simulink model "explore"  (Simulink 8.3)
settings: Solver=ode4  StartTime=0.0  StopTime=600  FixedStep=0.001  RelTol=1e-3
PostLoadFcn:
  | , if any(exist('dsrtsu_mdlpostloadfcn', 'file') == [2, 3, 6]), try dsrtsu_mdlpostloadfcn('Execute', bdroot); catch fprintf('Error in PostLoadFcn (dsrtsu_mdlpostloadfcn) for model "%s":\n %s\n', bdroot, lasterr); end, end,
values from neighbouring files (symbols this model uses):
  A = kron(eye(2),A)    [explore_setup.m]
  Ae = Ah    [explore_setup.m]
  Av = [0 1 0; zeros(2,1) Av]    [explore_setup.m]
  Aw = [0 1; 0 Aw]    [explore_setup.m]
  B = kron(eye(2),B)    [explore_setup.m]
  Be = Bh    [explore_setup.m]
  Bv = [0; Bv]    [explore_setup.m]
  Bw = [0; Bw*Cw]    [explore_setup.m]
  Ce = Ch    [explore_setup.m]
  Cv = [1 0 0]    [explore_setup.m]
  Cw = [1 0]    [explore_setup.m]
  dt = 0.15    [explore_setup.m]
  Fu = kron(eye(2), Fu)    [explore_setup.m]
  Fus = kron(eye(2), Fus)    [explore_setup.m]
  Fx = kron(eye(2),Fx)    [explore_setup.m]
  Fxf = 1e-6*eye(8)    [explore_setup.m]
  Fxs = kron(eye(2),Fxs)    [explore_setup.m]
  goal = [1.8750    1.5000]    [explore_setup.m]    (also in visualizeSim.m = u(169:170))
  homePos = [-2.5 -1]    [explore_setup.m]
  Le = place(Ae', Ce', -[3.1 3.0 3.2])'    [explore_setup.m]
  Lv = place(Av', Cv', -[3.1 3.0 3.2])'    [explore_setup.m]
  Lw = place(Aw', Cw', -[3.1 3.0])'    [explore_setup.m]
  nodeV0 = (1/.4)*sqrt((nodeX-goal(1)).*(nodeX-goal(1))+(nodeY-goal(2)).*(nodeY-goal(2)))    [explore_setup.m]
  nodeX = [goal(1); nodeX]    [explore_setup.m]
  nodeY = [goal(2); nodeY]    [explore_setup.m]
  obst = [-2.4950    1.5000    1.3750    2.0000 ... (first row only)    [explore_setup.m]    (also in visualizeSim.m = reshape(obstIn,4,nObst)')
  Q = diag([5 5 5 2 5 5 5 2])    [explore_setup.m]
  Qf = diag([5 5 5 2 5 5 5 2])    [explore_setup.m]
  R = diag([10 10])    [explore_setup.m]
  T = 16    [explore_setup.m]
undefined symbols (not defined in the file or in its folder): bd, bx, C, Ef_block, g, gt, H, hc, hcs, hp, hps, hx, hxs, P, Ps
undefined symbols (not defined in the file): Ed, ef, Exf, f, ff, Fp, Fpf, Fps, fs, q, qf, r
libraries: simulink x1
settings Model: DSRTSU_INTERNAL_RTI_VER=400  DSRTSU_INTERNAL_RTI_TYPE=rti1401  Creator=aeagr  LastModifiedBy=aeagr  BufferReuse=off
settings OptimizationCC: BlockReduction=off  OptimizeBlockIOStorage=off  BufferReuse=off  GlobalBufferReuse=off  ExpressionFolding=off  ExpressionDepthLimit=2147483647  LocalBlockOutputs=off  SimCompilerOptimization=On
settings DebuggingCC: FcnCallInpInsideContextMsg=UseLocalSettings
settings HardwareCC: ProdIntDivRoundTo=Zero  ProdEndianess=BigEndian  ProdHWDeviceType=Generic->Custom  TargetIntDivRoundTo=Zero  TargetEndianess=BigEndian  TargetHWDeviceType=Generic->Custom
settings RTWCC: ProcessScript=grt_make_rtw_hook
settings GRTTargetCC: CombineOutputUpdateFcns=on  GRTInterface=off

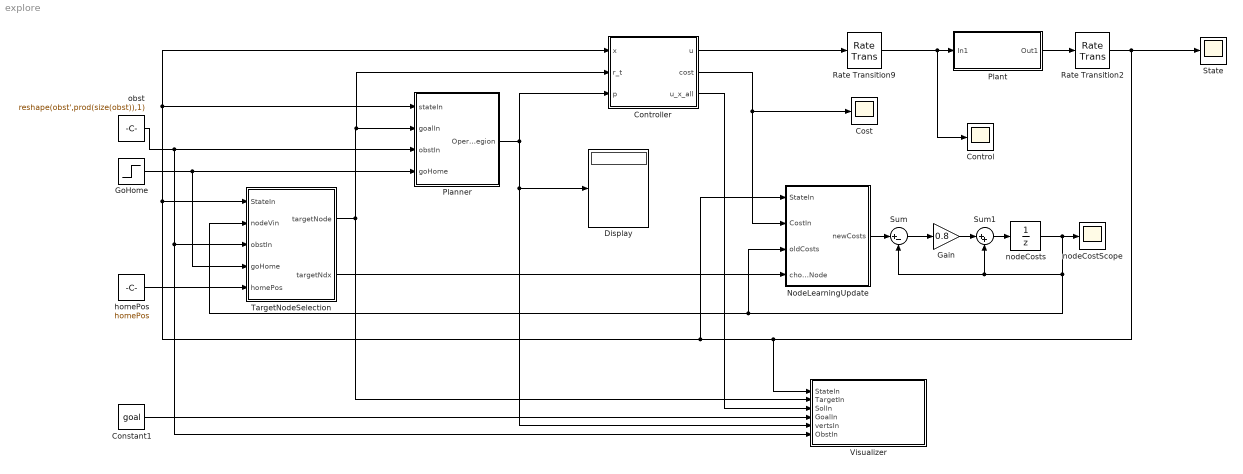
== system explore ==
  Constant1 : Constant  Value=goal
  Control : Scope
      settings: TimeRange=120  YMin=-0.05  YMax=0.12
  Controller : Subsystem  TreatAsAtomicUnit=on  SystemSampleTime=dt
  Cost : Scope
      settings: TimeRange=120  YMin=0  YMax=350  SaveName=ScopeData8
  Display : Display
  Gain : Gain  Gain=0.8
  GoHome : Step  Time=10  Before=1  After=0  SampleTime=dt
  NodeLearningUpdate : Subsystem  TreatAsAtomicUnit=on  SystemSampleTime=dt
  Planner : Subsystem  TreatAsAtomicUnit=on  SystemSampleTime=dt
  Plant : Subsystem
  Rate Transition2 : RateTransition  Integrity=off  OutPortSampleTimeOpt=Inherit  OutPortSampleTime=dt
  Rate Transition9 : RateTransition  Integrity=off  OutPortSampleTimeOpt=Inherit  OutPortSampleTime=dt
  State : Scope
      settings: TimeRange=60  YMin=-200  YMax=225
  Sum : Sum  Inputs=|+-
  Sum1 : Sum  Inputs=|++
  TargetNodeSelection : Subsystem  TreatAsAtomicUnit=on  SystemSampleTime=dt
  Visualizer : Subsystem
  homePos : Constant  Value=homePos
  nodeCostScope : Scope
      settings: TimeRange=120  YMin=0  YMax=19  SaveName=ScopeData2
  nodeCosts : UnitDelay  InitialCondition=nodeV0  SampleTime=dt
  obst : Constant  Value=reshape(obst',prod(size(obst)),1)
  wires:
  Plant/1(Out1) -> Rate Transition2/1
  Planner/1(Operating Region) -> Controller/3(p), Display/1, Visualizer/5(vertsIn)
  Controller/1(u) -> Rate Transition9/1
  Controller/3(u_x_all) -> Visualizer/3(SolIn)
  Constant1/1 -> Visualizer/4(GoalIn)
  obst/1 -> Planner/3(obstIn), Visualizer/6(ObstIn), TargetNodeSelection/3(obstIn)
  TargetNodeSelection/1(targetNode) -> Visualizer/2(TargetIn), Controller/2(r_t), Planner/2(goalIn)
  GoHome/1 -> TargetNodeSelection/4(goHome), Planner/4(goHome)
  Rate Transition9/1 -> Plant/1(In1), Control/1
  Controller/2(cost) -> NodeLearningUpdate/2(CostIn), Cost/1
  Rate Transition2/1 -> State/1, Visualizer/1(StateIn), NodeLearningUpdate/1(StateIn), TargetNodeSelection/1(StateIn), Controller/1(x), Planner/1(stateIn)
  TargetNodeSelection/2(targetNdx) -> NodeLearningUpdate/4(chosenNode)
  nodeCosts/1 -> nodeCostScope/1, TargetNodeSelection/2(nodeVin), NodeLearningUpdate/3(oldCosts), Sum1/2, Sum/2
  homePos/1 -> TargetNodeSelection/5(homePos)
  NodeLearningUpdate/1(newCosts) -> Sum/1
  Sum1/1 -> nodeCosts/1
  Sum/1 -> Gain/1
  Gain/1 -> Sum1/1

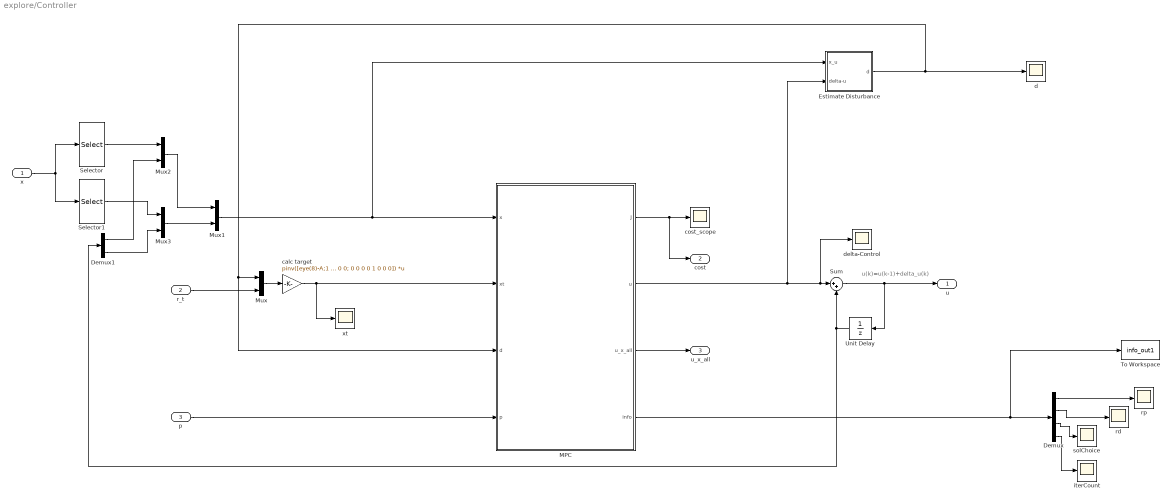
== system explore/Controller ==
  note: u(k)=u(k-1)+delta_u(k)
  x : Inport
  r_t : Inport  Port=2
  p : Inport  Port=3
  Demux : Demux
  Demux1 : Demux  Outputs=2
  Estimate Disturbance : Subsystem
  MPC : Subsystem  TreatAsAtomicUnit=on  mask{A=A, B=B, T=T, dt=-1, Q=Q, R=R, Qf=Qf, qv=q, rv=r, qfv=qf, Fx=Fx, Fu=Fu, Fp=Fp, f=f, Fxs=Fxs, Fus=Fus, Fps=Fps, fs=fs, Fxf=Fxf, Fpf=Fpf, ff=ff, Ef=Exf, Ed=Ed, e=ef, consAllBox=on, numNewton=4, kappa=0.005}
      mask prompts: T "Horizon length T"; dt "Time step"; qv "q"; rv "r"; qfv "qf"; e "ef"; consAllBox "Box constraints"; numNewton "Number of Newton Iterations"; kappa "Barrier weight kappa"
      mask init:
      | % build the big matrices
      | [H,g,gt,P,hx,hc,C,bx,bd,Ps,hxs,hcs,Ef_block,Ed_block,ef_block,hp,hps] = buildmatrices(A,B,Q,R,qv,rv,Qf,qfv,T,Fx,Fu,f,Fxs,Fus,fs,Fxf,ff,Ef,e,Ed,Fp,Fps,Fpf);
      | 
      | % options
      | opts=[];
      | disp(consAllBox)
      | if consAllBox,
      |     opts(1)=1; % 1 = assume diagonal Phi when solving
      | else
      |     opts(1)=0;
      | end
      | opts(2)=numNewton; % Newton iterations
      | opts(3)=1; % 1 = use soft constraints
      | opts(4)=0; % 1 = checking on
      | opts(7)=kappa; % tuning of barrier weight kappa
  Mux{,1..3} (4 alike) : Mux  Inputs=2
  Selector : Selector  InputPortWidth=6  Indices=[1 2 3]
  Selector1 : Selector  InputPortWidth=6  Indices=[1 2 3]+3
  Sum : Sum  Inputs=|++
  To Workspace : ToWorkspace  VariableName=info_out1  SampleTime=-1
  Unit Delay : UnitDelay  SampleTime=-1
  calc target : Gain  Gain=pinv([eye(8)-A;1 0 0 0 0 0 0 0; 0 0 0 0 1 0 0 0])  Multiplication=Matrix(K*u)
  cost_scope : Scope
      settings: YMin=-0.25  YMax=2.5  SaveName=ScopeData10
  d : Scope
      settings: YMin=-0.00025  YMax=0.002  SaveName=ScopeData11
  delta-Control : Scope
      settings: TimeRange=240  YMin=-0.4  YMax=0.35  SaveName=ScopeData2
  iterCount : Scope
      settings: TimeRange=200  YMin=0  YMax=25  SaveName=ScopeData12
  rd : Scope
      settings: YMin=0  YMax=13  SaveName=ScopeData13
  rp : Scope
      settings: YMin=1.65436e-24  YMax=2.75e-08  SaveName=ScopeData14
  solChoice : Scope
      settings: YMin=0.95  YMax=1.05  SaveName=ScopeData15
  xt : Scope
      settings: YMin=-0.25  YMax=2.5  SaveName=ScopeData16
  u : Outport
  cost : Outport  Port=2
  u_x_all : Outport  Port=3
  wires:
  Sum/1 -> u/1, Unit Delay/1
  MPC/2(u) -> Sum/1, delta-Control/1, Estimate Disturbance/2(delta-u)
  Unit Delay/1 -> Demux1/1, Sum/2
  Mux1/1 -> MPC/1(x), Estimate Disturbance/1(x_u)
  Demux/1 -> rp/1
  Demux/2 -> rd/1
  Demux/3 -> solChoice/1
  Estimate Disturbance/1(d) -> MPC/3(d), Mux/1, d/1
  Mux/1 -> calc target/1
  r_t/1 -> Mux/2
  calc target/1 -> MPC/2(xt), xt/1
  Demux/4 -> iterCount/1
  MPC/4(info) -> To Workspace/1, Demux/1
  p/1 -> MPC/4(p)
  MPC/1(J) -> cost/1, cost_scope/1
  MPC/3(u_x_all) -> u_x_all/1
  x/1 -> Selector1/1, Selector/1
  Selector/1 -> Mux2/1
  Selector1/1 -> Mux3/1
  Demux1/1 -> Mux2/2
  Demux1/2 -> Mux3/2
  Mux3/1 -> Mux1/2
  Mux2/1 -> Mux1/1

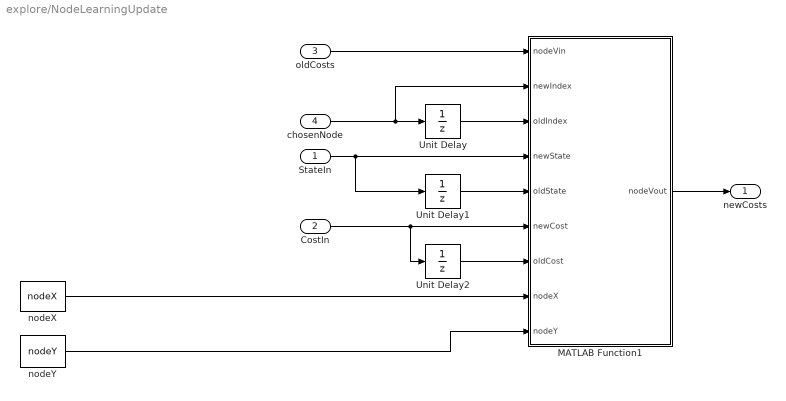
== system explore/NodeLearningUpdate ==
  StateIn : Inport
  CostIn : Inport  Port=2
  oldCosts : Inport  Port=3
  chosenNode : Inport  Port=4
  MATLAB Function1 : MATLAB Function  TreatAsAtomicUnit=on
  Unit Delay : UnitDelay  SampleTime=-1
  Unit Delay1 : UnitDelay  SampleTime=-1
  Unit Delay2 : UnitDelay  SampleTime=-1
  nodeX : Constant  Value=nodeX
  nodeY : Constant  Value=nodeY
  newCosts : Outport
  wires:
  CostIn/1 -> Unit Delay2/1, MATLAB Function1/6(newCost)
  StateIn/1 -> MATLAB Function1/4(newState), Unit Delay1/1
  nodeY/1 -> MATLAB Function1/9(nodeY)
  nodeX/1 -> MATLAB Function1/8(nodeX)
  Unit Delay2/1 -> MATLAB Function1/7(oldCost)
  Unit Delay1/1 -> MATLAB Function1/5(oldState)
  chosenNode/1 -> MATLAB Function1/2(newIndex), Unit Delay/1
  Unit Delay/1 -> MATLAB Function1/3(oldIndex)
  MATLAB Function1/1(nodeVout) -> newCosts/1
  oldCosts/1 -> MATLAB Function1/1(nodeVin)

== system explore/Planner ==
  stateIn : Inport
  goalIn : Inport  Port=2
  obstIn : Inport  Port=3
  goHome : Inport  Port=4
  MATLAB Function : MATLAB Function  TreatAsAtomicUnit=on
  Operating Region : Outport
  wires:
  stateIn/1 -> MATLAB Function/1(state)
  goHome/1 -> MATLAB Function/2(goHome)
  MATLAB Function/1(verts) -> Operating Region/1
  goalIn/1 -> MATLAB Function/4(goal)
  obstIn/1 -> MATLAB Function/3(obst)

== system explore/Plant ==
  In1 : Inport
  AR.Drone : Subsystem
  Demux1 : Demux  Outputs=2
  Fixed point hold : Subsystem
  Mux : Mux  Inputs=3
  Other inputs : Selector  InputPortWidth=4  Indices=[3 4]
  "Position, Velocity" : Selector  InputPortWidth=11  Indices=[1 4 7 10 2 5 8 11]
  Select Gxy : Selector  InputPortWidth=11  Indices=[1 2 3 4 5 6]
  Out1 : Outport
  wires:
  Other inputs/1 -> Demux1/1
  Mux/1 -> AR.Drone/1(U Global)
  Fixed point hold/1(U Global) -> Other inputs/1
  "Position, Velocity"/1 -> Fixed point hold/1(X Global)
  AR.Drone/1(X Global) -> "Position, Velocity"/1, Select Gxy/1
  Select Gxy/1 -> Out1/1
  In1/1 -> Mux/1
  Demux1/1 -> Mux/2
  Demux1/2 -> Mux/3

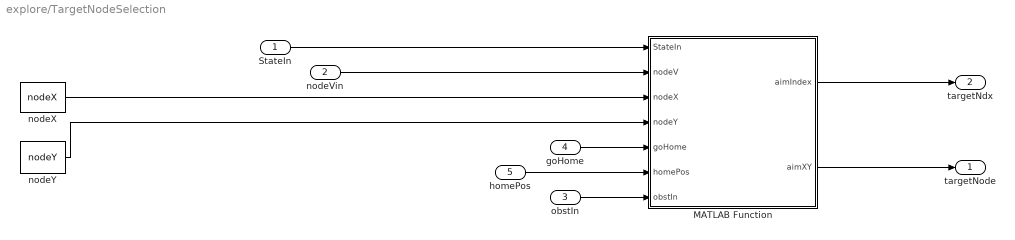
== system explore/TargetNodeSelection ==
  StateIn : Inport
  nodeVin : Inport  Port=2
  obstIn : Inport  Port=3
  goHome : Inport  Port=4
  homePos : Inport  Port=5
  MATLAB Function : MATLAB Function  TreatAsAtomicUnit=on  SystemSampleTime=dt
  nodeX : Constant  Value=nodeX
  nodeY : Constant  Value=nodeY
  targetNode : Outport
  targetNdx : Outport  Port=2
  wires:
  nodeX/1 -> MATLAB Function/3(nodeX)
  nodeY/1 -> MATLAB Function/4(nodeY)
  StateIn/1 -> MATLAB Function/1(StateIn)
  MATLAB Function/2(aimXY) -> targetNode/1
  goHome/1 -> MATLAB Function/5(goHome)
  obstIn/1 -> MATLAB Function/7(obstIn)
  MATLAB Function/1(aimIndex) -> targetNdx/1
  nodeVin/1 -> MATLAB Function/2(nodeV)
  homePos/1 -> MATLAB Function/6(homePos)

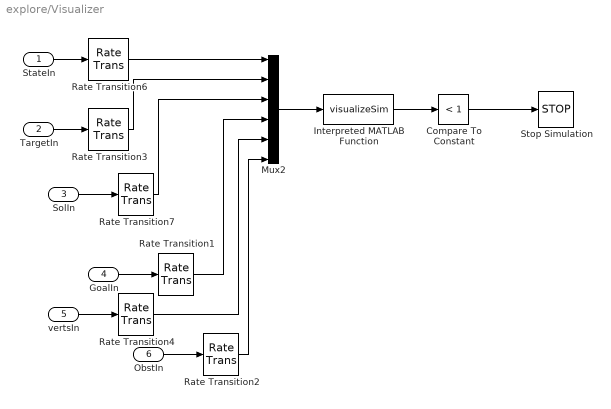
== system explore/Visualizer ==
  StateIn : Inport
  TargetIn : Inport  Port=2
  SolIn : Inport  Port=3
  GoalIn : Inport  Port=4
  vertsIn : Inport  Port=5
  ObstIn : Inport  Port=6
  Compare To Constant : simulink/Logic and Bit Operations/Compare To Constant  relop=<  const=1  OutDataTypeStr=boolean
  Interpreted MATLAB Function : MATLABFcn  MATLABFcn=visualizeSim
  Mux2 : Mux  Inputs=6
  Rate Transition{1..4,6..7} (6 alike) : RateTransition  Integrity=off  OutPortSampleTime=dt
  Stop Simulation : Stop
  wires:
  Interpreted MATLAB Function/1 -> Compare To Constant/1
  Mux2/1 -> Interpreted MATLAB Function/1
  Rate Transition6/1 -> Mux2/1
  Rate Transition3/1 -> Mux2/2
  Rate Transition7/1 -> Mux2/3
  StateIn/1 -> Rate Transition6/1
  TargetIn/1 -> Rate Transition3/1
  SolIn/1 -> Rate Transition7/1
  GoalIn/1 -> Rate Transition1/1
  ObstIn/1 -> Rate Transition2/1
  Rate Transition1/1 -> Mux2/4
  Rate Transition2/1 -> Mux2/6
  vertsIn/1 -> Rate Transition4/1
  Rate Transition4/1 -> Mux2/5
  Compare To Constant/1 -> Stop Simulation/1

== system explore/Controller/Estimate Disturbance ==
  x_u : Inport
  delta-u : Inport  Port=2
  A : Gain  Gain=A  Multiplication=Matrix(K*u)
  Add2 : Sum
  Add3 : Sum  Inputs=+-
  B : Gain  Gain=B  Multiplication=Matrix(K*u)
  Discrete Transfer Fcn : DiscreteTransferFcn  Numerator=[0.5]  Denominator=[1 -0.5]
  Unit Delay : UnitDelay  SampleTime=-1
  Unit Delay1 : UnitDelay  SampleTime=-1
  d : Outport
  wires:
  Unit Delay1/1 -> A/1
  Unit Delay/1 -> B/1
  A/1 -> Add2/1
  B/1 -> Add2/2
  Add2/1 -> Add3/2
  x_u/1 -> Unit Delay1/1, Add3/1
  delta-u/1 -> Unit Delay/1
  Add3/1 -> Discrete Transfer Fcn/1
  Discrete Transfer Fcn/1 -> d/1

== system explore/Controller/MPC ==
  x : Inport
  xt : Inport  Port=2
  d : Inport  Port=3
  p : Inport  Port=4
  Subsystem : Subsystem  TreatAsAtomicUnit=on  SystemSampleTime=dt
  J : Outport
  u : Outport  Port=2
  u_x_all : Outport  Port=3
  info : Outport  Port=4
  wires:
  x/1 -> Subsystem/1(In1)
  xt/1 -> Subsystem/2(In2)
  d/1 -> Subsystem/3(In3)
  p/1 -> Subsystem/4(In4)
  Subsystem/1(Cost) -> J/1
  Subsystem/2(u) -> u/1
  Subsystem/4(info) -> info/1
  Subsystem/3(u_x_all) -> u_x_all/1

== system explore/Plant/AR.Drone ==
  U Global : Inport
  Constant : Constant  Value=zeros(4,1)
  Constant1 : Constant  Value=0
  Saturation : Saturate  UpperLimit=[0.37 0.37 1 1]  LowerLimit=-[0.37 0.37 1 1]
  State Estimator : Subsystem
  To Metres : Gain  Gain=[1e-3 1e-3 1e-3 1]
  X Global : Outport
  wires:
  U Global/1 -> Saturation/1
  To Metres/1 -> State Estimator/1(Y Global)
  State Estimator/1(X Global) -> X Global/1
  Saturation/1 -> State Estimator/2(U Global)
  Constant1/1 -> State Estimator/3(Valid State)
  Constant/1 -> To Metres/1

== system explore/Plant/Fixed point hold ==
  X Global : Inport
  Add : Sum
  Error : Sum  Inputs=-+
  Gain Position : Gain  Gain=[0.5 0.5 1.2 1]'
  Gain Velocity : Gain  Gain=[0.3 0.3 0.4 0]'
  Position : Selector  InputPortWidth=8  Indices=[1 2 3 4]
  Reference Point : Constant  Value=[0 0 1 -pi/2 0 0 0 0]'
  Velocity : Selector  InputPortWidth=8  Indices=[5 6 7 8]
  U Global : Outport
  wires:
  Gain Velocity/1 -> Add/2
  Gain Position/1 -> Add/1
  X Global/1 -> Error/1
  Reference Point/1 -> Error/2
  Add/1 -> U Global/1
  Position/1 -> Gain Position/1
  Velocity/1 -> Gain Velocity/1
  Error/1 -> Position/1, Velocity/1

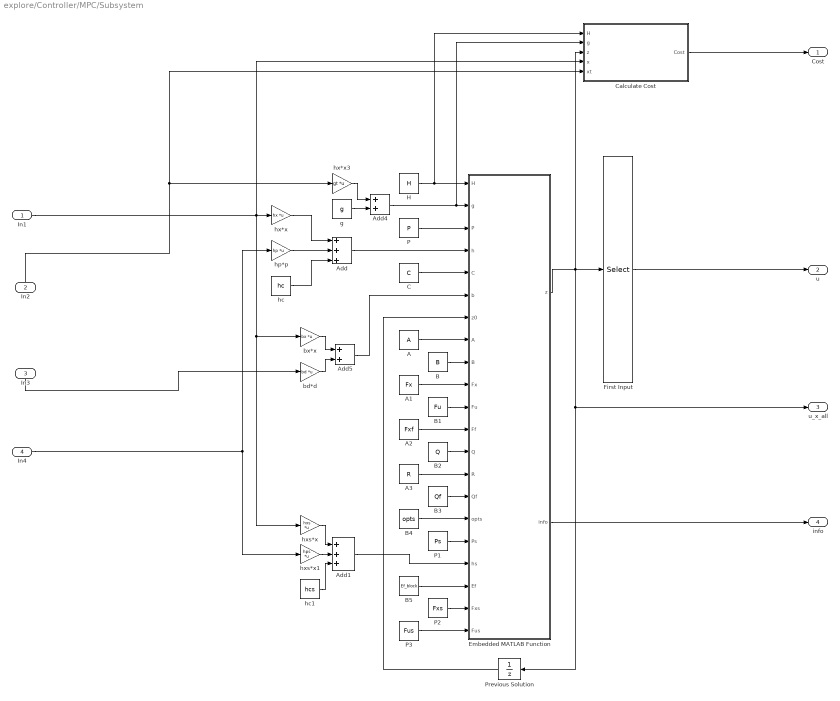
== system explore/Controller/MPC/Subsystem ==
  In1 : Inport
  In2 : Inport  Port=2
  In3 : Inport  Port=3
  In4 : Inport  Port=4
  A : Constant  Value=A
  A1 : Constant  Value=Fx
  A2 : Constant  Value=Fxf
  A3 : Constant  Value=R
  Add : Sum  Inputs=+++
  Add1 : Sum  Inputs=+++
  Add4 : Sum
  Add5 : Sum
  B : Constant  Value=B
  B1 : Constant  Value=Fu
  B2 : Constant  Value=Q
  B3 : Constant  Value=Qf
  B4 : Constant  Value=opts
  B5 : Constant  Value=Ef_block
  C : Constant  Value=C
  Calculate Cost : Subsystem
  Embedded MATLAB Function : MATLAB Function  TreatAsAtomicUnit=on
      settings: RTWFileNameOpts=Use subsystem name
  First Input : Selector  InputPortWidth=size(H,1)  Indices=1:size(B,2)
  H : Constant  Value=H
  P : Constant  Value=P
  P1 : Constant  Value=Ps
  P2 : Constant  Value=Fxs
  P3 : Constant  Value=Fus
  Previous Solution : UnitDelay  SampleTime=-1
  bd*d : Gain  Gain=bd  Multiplication=Matrix(K*u)
  bx*x : Gain  Gain=bx  Multiplication=Matrix(K*u)
  g : Constant  Value=g
  hc : Constant  Value=hc
  hc1 : Constant  Value=hcs
  hp*p : Gain  Gain=hp  Multiplication=Matrix(K*u)
  hx*x : Gain  Gain=hx  Multiplication=Matrix(K*u)
  hx*x3 : Gain  Gain=gt  Multiplication=Matrix(K*u)
  hxs*x : Gain  Gain=hxs  Multiplication=Matrix(K*u)
  hxs*x1 : Gain  Gain=hps  Multiplication=Matrix(K*u)
  Cost : Outport
  u : Outport  Port=2
  u_x_all : Outport  Port=3
  info : Outport  Port=4
  wires:
  H/1 -> Embedded MATLAB Function/1(H), Calculate Cost/1(H)
  Embedded MATLAB Function/1(z) -> u_x_all/1, Previous Solution/1, First Input/1, Calculate Cost/3(z)
  Previous Solution/1 -> Embedded MATLAB Function/7(z0)
  B/1 -> Embedded MATLAB Function/9(B)
  hx*x/1 -> Add/1
  Add/1 -> Embedded MATLAB Function/4(h)
  A3/1 -> Embedded MATLAB Function/14(R)
  P/1 -> Embedded MATLAB Function/3(P)
  C/1 -> Embedded MATLAB Function/5(C)
  B3/1 -> Embedded MATLAB Function/15(Qf)
  A/1 -> Embedded MATLAB Function/8(A)
  First Input/1 -> u/1
  In2/1 -> Calculate Cost/5(xt), hx*x3/1
  In3/1 -> bd*d/1
  In1/1 -> Calculate Cost/4(x), bx*x/1, hxs*x/1, hx*x/1
  A2/1 -> Embedded MATLAB Function/12(Ff)
  g/1 -> Add4/2
  P2/1 -> Embedded MATLAB Function/20(Fxs)
  Embedded MATLAB Function/2(info) -> info/1
  In4/1 -> hp*p/1, hxs*x1/1
  Add1/1 -> Embedded MATLAB Function/18(hs)
  A1/1 -> Embedded MATLAB Function/10(Fx)
  bx*x/1 -> Add5/1
  hxs*x/1 -> Add1/1
  Add4/1 -> Embedded MATLAB Function/2(g), Calculate Cost/2(g)
  B1/1 -> Embedded MATLAB Function/11(Fu)
  hx*x3/1 -> Add4/1
  hp*p/1 -> Add/2
  hxs*x1/1 -> Add1/2
  hc1/1 -> Add1/3
  P3/1 -> Embedded MATLAB Function/21(Fus)
  B5/1 -> Embedded MATLAB Function/19(Ef)
  P1/1 -> Embedded MATLAB Function/17(Ps)
  hc/1 -> Add/3
  bd*d/1 -> Add5/2
  Add5/1 -> Embedded MATLAB Function/6(b)
  B4/1 -> Embedded MATLAB Function/16(opts)
  B2/1 -> Embedded MATLAB Function/13(Q)
  Calculate Cost/1(Cost) -> Cost/1

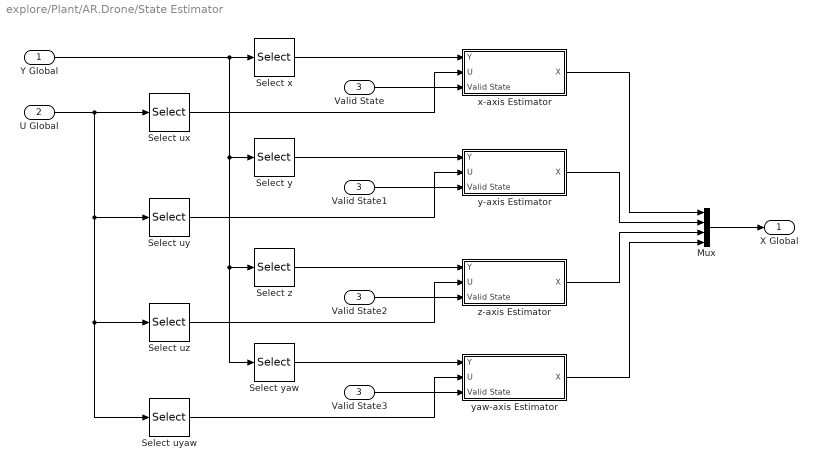
== system explore/Plant/AR.Drone/State Estimator ==
  Y Global : Inport
  U Global : Inport  Port=2
  Valid State : Inport  Port=3
  Mux : Mux
  Select ux : Selector  InputPortWidth=4
  Select uy : Selector  InputPortWidth=4  Indices=2
  Select uyaw : Selector  InputPortWidth=4  Indices=4
  Select uz : Selector  InputPortWidth=4  Indices=3
  Select x : Selector
  Select y : Selector  Indices=2
  Select yaw : Selector  Indices=4
  Select z : Selector  Indices=[3]
  Valid State1 : InportShadow  Port=3
  Valid State2 : InportShadow  Port=3
  Valid State3 : InportShadow  Port=3
  x-axis Estimator : Subsystem
  y-axis Estimator : Subsystem
  yaw-axis Estimator : Subsystem
  z-axis Estimator : Subsystem
  X Global : Outport
  wires:
  Y Global/1 -> Select x/1, Select y/1, Select yaw/1, Select z/1
  Select x/1 -> x-axis Estimator/1(Y)
  Select y/1 -> y-axis Estimator/1(Y)
  Select yaw/1 -> yaw-axis Estimator/1(Y)
  Select ux/1 -> x-axis Estimator/2(U)
  Select uy/1 -> y-axis Estimator/2(U)
  Select uyaw/1 -> yaw-axis Estimator/2(U)
  U Global/1 -> Select ux/1, Select uy/1, Select uyaw/1, Select uz/1
  Select z/1 -> z-axis Estimator/1(Y)
  Select uz/1 -> z-axis Estimator/2(U)
  Mux/1 -> X Global/1
  x-axis Estimator/1(X) -> Mux/1
  y-axis Estimator/1(X) -> Mux/2
  z-axis Estimator/1(X) -> Mux/3
  yaw-axis Estimator/1(X) -> Mux/4
  Valid State/1 -> x-axis Estimator/3(Valid State)
  Valid State1/1 -> y-axis Estimator/3(Valid State)
  Valid State3/1 -> yaw-axis Estimator/3(Valid State)
  Valid State2/1 -> z-axis Estimator/3(Valid State)

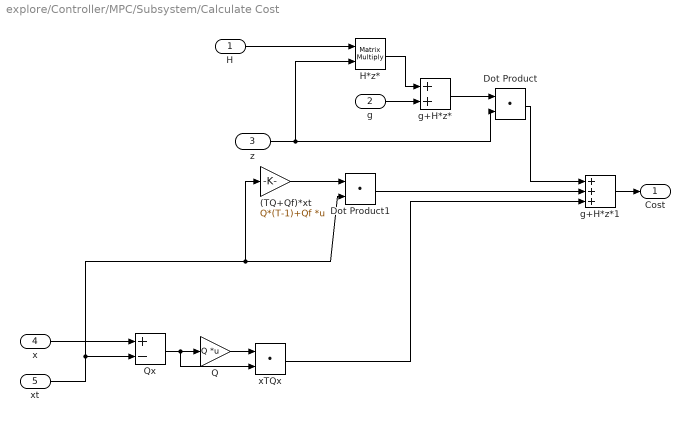
== system explore/Controller/MPC/Subsystem/Calculate Cost ==
  H : Inport
  g : Inport  Port=2
  z : Inport  Port=3
  x : Inport  Port=4
  xt : Inport  Port=5
  (TQ+Qf)*xt : Gain  Gain=Q*(T-1)+Qf  Multiplication=Matrix(K*u)
  Dot Product : DotProduct  InputSameDT=on  OutDataTypeStr=Inherit: Inherit via internal rule
  Dot Product1 : DotProduct  InputSameDT=on  OutDataTypeStr=Inherit: Inherit via internal rule
  H*z* : Product  Multiplication=Matrix(*)  RndMeth=Zero
  Q : Gain  Gain=Q  Multiplication=Matrix(K*u)
  Qx : Sum  Inputs=+-
  g+H*z* : Sum
  g+H*z*1 : Sum  Inputs=+++
  xTQx : DotProduct  InputSameDT=on  OutDataTypeStr=Inherit: Inherit via internal rule
  Cost : Outport
  wires:
  H*z*/1 -> g+H*z*/1
  g+H*z*/1 -> Dot Product/1
  (TQ+Qf)*xt/1 -> Dot Product1/1
  Dot Product/1 -> g+H*z*1/1
  Dot Product1/1 -> g+H*z*1/2
  Qx/1 -> Q/1, xTQx/2
  Q/1 -> xTQx/1
  xTQx/1 -> g+H*z*1/3
  H/1 -> H*z*/1
  g/1 -> g+H*z*/2
  z/1 -> H*z*/2, Dot Product/2
  x/1 -> Qx/1
  xt/1 -> Qx/2, (TQ+Qf)*xt/1, Dot Product1/2
  g+H*z*1/1 -> Cost/1

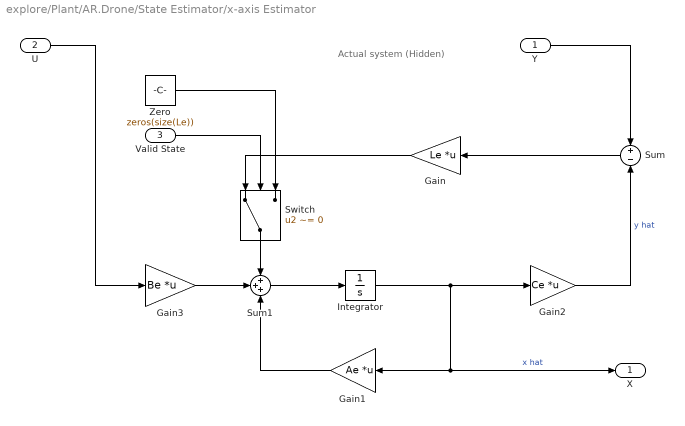
== system explore/Plant/AR.Drone/State Estimator/x-axis Estimator ==
  note: Actual system (Hidden)
  Y : Inport
  U : Inport  Port=2
  Valid State : Inport  Port=3
  Gain : Gain  Gain=Le  Multiplication=Matrix(K*u)
  Gain1 : Gain  Gain=Ae  Multiplication=Matrix(K*u)
  Gain2 : Gain  Gain=Ce  Multiplication=Matrix(K*u)
  Gain3 : Gain  Gain=Be  Multiplication=Matrix(K*u)
  Integrator : Integrator
  Sum : Sum  Inputs=+|-
  Sum1 : Sum  Inputs=+++
  Switch : Switch  Criteria=u2 ~= 0
  Zero : Constant  Value=zeros(size(Le))
  X : Outport
  wires:
  U/1 -> Gain3/1
  Y/1 -> Sum/1
  Sum/1 -> Gain/1
  Sum1/1 -> Integrator/1
  Gain1/1 -> Sum1/3
  Integrator/1 -> Gain2/1, Gain1/1, X/1  "x hat"
  Gain2/1 -> Sum/2  "y hat"
  Gain3/1 -> Sum1/2
  Valid State/1 -> Switch/2
  Gain/1 -> Switch/1
  Switch/1 -> Sum1/1
  Zero/1 -> Switch/3

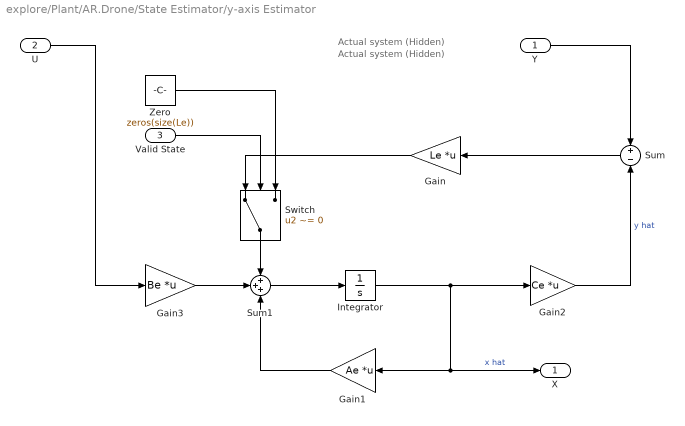
== system explore/Plant/AR.Drone/State Estimator/y-axis Estimator ==
  note: Actual system (Hidden)
  note: Actual system (Hidden)
  Y : Inport
  U : Inport  Port=2
  Valid State : Inport  Port=3
  Gain : Gain  Gain=Le  Multiplication=Matrix(K*u)
  Gain1 : Gain  Gain=Ae  Multiplication=Matrix(K*u)
  Gain2 : Gain  Gain=Ce  Multiplication=Matrix(K*u)
  Gain3 : Gain  Gain=Be  Multiplication=Matrix(K*u)
  Integrator : Integrator
  Sum : Sum  Inputs=+|-
  Sum1 : Sum  Inputs=+++
  Switch : Switch  Criteria=u2 ~= 0
  Zero : Constant  Value=zeros(size(Le))
  X : Outport
  wires:
  Gain3/1 -> Sum1/2
  Gain2/1 -> Sum/2  "y hat"
  Integrator/1 -> Gain2/1, Gain1/1, X/1  "x hat"
  Gain1/1 -> Sum1/3
  Sum1/1 -> Integrator/1
  Sum/1 -> Gain/1
  Y/1 -> Sum/1
  U/1 -> Gain3/1
  Valid State/1 -> Switch/2
  Gain/1 -> Switch/1
  Switch/1 -> Sum1/1
  Zero/1 -> Switch/3

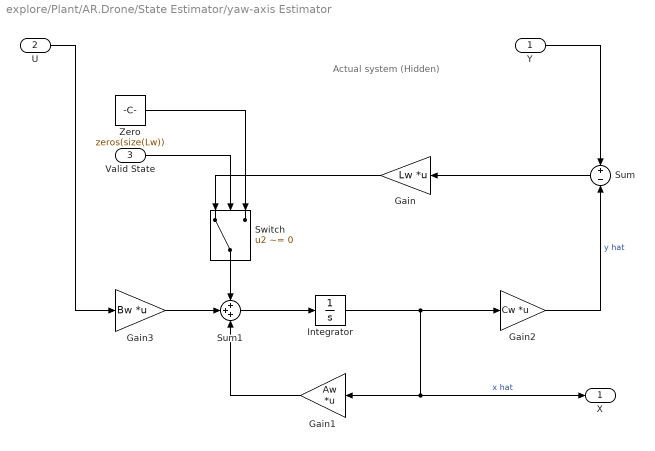
== system explore/Plant/AR.Drone/State Estimator/yaw-axis Estimator ==
  note: Actual system (Hidden)
  Y : Inport
  U : Inport  Port=2
  Valid State : Inport  Port=3
  Gain : Gain  Gain=Lw  Multiplication=Matrix(K*u)
  Gain1 : Gain  Gain=Aw  Multiplication=Matrix(K*u)
  Gain2 : Gain  Gain=Cw  Multiplication=Matrix(K*u)
  Gain3 : Gain  Gain=Bw  Multiplication=Matrix(K*u)
  Integrator : Integrator
  Sum : Sum  Inputs=+|-
  Sum1 : Sum  Inputs=+++
  Switch : Switch  Criteria=u2 ~= 0
  Zero : Constant  Value=zeros(size(Lw))
  X : Outport
  wires:
  Gain3/1 -> Sum1/2
  Gain2/1 -> Sum/2  "y hat"
  Integrator/1 -> Gain1/1, X/1, Gain2/1  "x hat"
  Gain1/1 -> Sum1/3
  Sum1/1 -> Integrator/1
  Sum/1 -> Gain/1
  Y/1 -> Sum/1
  U/1 -> Gain3/1
  Valid State/1 -> Switch/2
  Gain/1 -> Switch/1
  Switch/1 -> Sum1/1
  Zero/1 -> Switch/3

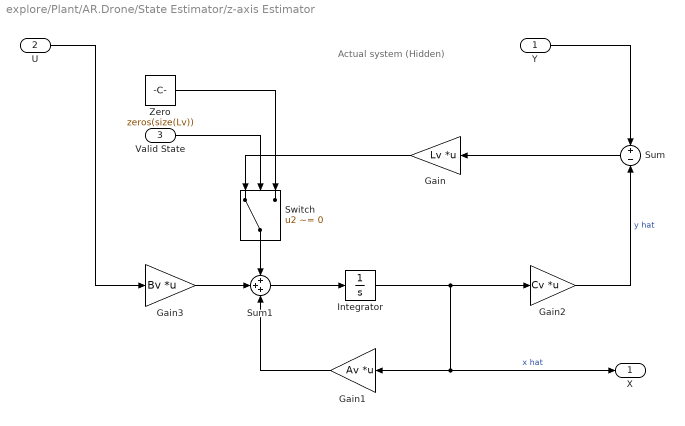
== system explore/Plant/AR.Drone/State Estimator/z-axis Estimator ==
  note: Actual system (Hidden)
  Y : Inport
  U : Inport  Port=2
  Valid State : Inport  Port=3
  Gain : Gain  Gain=Lv  Multiplication=Matrix(K*u)
  Gain1 : Gain  Gain=Av  Multiplication=Matrix(K*u)
  Gain2 : Gain  Gain=Cv  Multiplication=Matrix(K*u)
  Gain3 : Gain  Gain=Bv  Multiplication=Matrix(K*u)
  Integrator : Integrator
  Sum : Sum  Inputs=+|-
  Sum1 : Sum  Inputs=+++
  Switch : Switch  Criteria=u2 ~= 0
  Zero : Constant  Value=zeros(size(Lv))
  X : Outport
  wires:
  U/1 -> Gain3/1
  Y/1 -> Sum/1
  Sum/1 -> Gain/1
  Sum1/1 -> Integrator/1
  Gain1/1 -> Sum1/3
  Integrator/1 -> Gain2/1, Gain1/1, X/1  "x hat"
  Gain2/1 -> Sum/2  "y hat"
  Gain3/1 -> Sum1/2
  Valid State/1 -> Switch/2
  Gain/1 -> Switch/1
  Switch/1 -> Sum1/1
  Zero/1 -> Switch/3

== matlab function TargetNodeSelection/MATLAB Function ==
  data: StateIn input double; aimIndex output double; nodeV input double; nodeX input double; nodeY input double; aimXY output double; goHome input double; homePos input double; obstIn input double
function [aimIndex,aimXY] = chooseAiming(StateIn,nodeV,nodeX,nodeY,goHome,homePos,obstIn)
%#codegen

% number of nodes
nNodes = length(nodeV);

% characteristic velocity
v = 0.4;

% cost of choosing node from here
choiceCosts = nodeV + sqrt((nodeX-StateIn(1)).*(nodeX-StateIn(1)) + (nodeY-StateIn(4)).*(nodeY-StateIn(4)))/v;

% obstacle enlargement tolerance
dObst = 0.25;

if goHome>0,
    
    % start of sim, just go towards start point
    aimXY = homePos;
    aimIndex = 0;
    
else,
    
    % number of obstacles
    nObst = floor(length(obstIn)/4);
    % reshape obstacles into matrix
    obst = reshape(obstIn,4,nObst)';
    % enlarge for vehicle size
    obst(:,[1 3]) = obst(:,[1 3]) - dObst;
    obst(:,[2 4]) = obst(:,[2 4]) + dObst;
    
    % check visibility of nodes - assume true to begin
    nodeVis = true(nNodes,1);
    
    % loop through each
    for nn=1:nNodes,
        
        % check against each obstacle
        for kk=1:nObst,
            
            % if inside,
            if (nodeX(nn)>obst(kk,1))&&(nodeX(nn)<obst(kk,2))&&(nodeY(nn)>obst(kk,3))&&(nodeY(nn)<obst(kk,4)),
                nodeVis(nn)=false;
                break
            end
            
            % not inside, so check visibility
            if linesIntersect([nodeX(nn);nodeY(nn)],[StateIn(1);StateIn(4)],[obst(kk,1);obst(kk,3)],[obst(kk,2);obst(kk,4)])>1,
                nodeVis(nn)=false;
                break
            end
            % and against other side
            if linesIntersect([nodeX(nn);nodeY(nn)],[StateIn(1);StateIn(4)],[obst(kk,2);obst(kk,3)],[obst(kk,1);obst(kk,4)])>1,
                nodeVis(nn)=false;
                break
            end
            
        end
        
    end
    
    % always choose target if it's visible
    if nodeVis(1),
        
        aimIndex=1;
        
    else
        
        % list form
        visNodeList = find(nodeVis);
        
        % find node with lowest cost-to-go
        [minV,visIndex]=min(choiceCosts(visNodeList));
        
        % find index in original list
        aimIndex = visNodeList(visIndex);
        
    end
    
    % debug - take'em all
    %[minV,aimIndex]=min(nodeV);
    
    % find its coordinates
    aimXY = [nodeX(aimIndex); nodeY(aimIndex)];
    
end

== matlab function Controller/MPC/Subsystem/Embedded MATLAB Function ==
  data: H input double; z output double; g input double; P input double; h input double; C input double; b input double size=size(C,1); z0 input double; A input double; B input double; Fx input double; Fu input double; Ff input double; Q input double; R input double; Qf input double; info output double; opts input double; Ps input double; hs input double; Ef input double; Fxs input double; Fus input double
function [z,info] = mpcsolve_simk(H,g,P,h,C,b,z0,A,B,Fx,Fu,Ff,Q,R,Qf,opts,Ps,hs,Ef,Fxs,Fus)
%#codegen

% just call to the Matlab version
[z,info] = mpcsolve(H,g,P,h,C,b,z0,A,B,Fx,Fu,Ff,Q,R,Qf,opts,Ps,hs,Ef,Fxs,Fus);

== matlab function Planner/MATLAB Function ==
  data: state input double; goHome input double; verts output double; obst input double; goal input double
function verts  = fcn(state, goHome,obst,goal)
% %#codegen

% Set point is the target
%  - Has six states, [x x' x'' y y'' y'']
%  - Position between [0, 1]
% verts gives the valid operating region, i.e. for obstacle avoidance
% verts format is [xmin xmax ymin ymax]

% Current position
posn = state([1 4])';

% number of obstacles
nObst = floor(length(obst)/4);

% Obstacle format: [xmin xmax ymin ymax]
obst = reshape(obst,4,nObst)';

% Expand the obstacles, for safety
obst(:,[1 3]) = obst(:,[1 3]) - 0.25;
obst(:,[2 4]) = obst(:,[2 4]) + 0.25;

% default box size
defBox = 1;

% default box is centred on current
verts = [posn(1)-defBox posn(1)+defBox posn(2)-defBox posn(2)+defBox]';

% if not going home
if goHome<1,
    
    % work through each obstacle
    for kk=1:nObst,
        
        % skip it if no overlap
        if obst(kk,2)<=verts(1),
            continue
        end
        if obst(kk,1)>=verts(2),
            continue
        end
        if obst(kk,4)<=verts(3),
            continue
        end
        if obst(kk,3)>=verts(4),
            continue
        end
        
        % find incursions
        incs = [obst(kk,2)-verts(1);
                verts(2)-obst(kk,1);
                obst(kk,4)-verts(3);
                verts(4)-obst(kk,3)];
            
        % interested in smallest positive incursion, so knock out the
        % negative ones
        incs = incs + 1000*defBox*(incs<=0);
            
        % pick the smallest
        [mininc,idxinc]=min(incs);                
        
        % modify vertices
        switch idxinc,            
            case 1
                verts(1)=obst(kk,2);
            case 2
                verts(2)=obst(kk,1);
            case 3
                verts(3)=obst(kk,4);
            case 4
                verts(4)=obst(kk,3);
        end
        
    end
    
end

== matlab function NodeLearningUpdate/MATLAB Function1 ==
  data: nodeVin input double; nodeVout output double; newIndex input double; oldIndex input double; newState input double; oldState input double; newCost input double; oldCost input double; nodeX input double; nodeY input double
function nodeVout  = learningUpdate(nodeVin,newIndex,oldIndex,newState,oldState,newCost,oldCost,nodeX,nodeY)
%#codegen

% default - no change
nodeVout = nodeVin;

% only update if new state is something
% and if old index was not goal
if (newIndex>0) && (oldIndex>1)

    % just need positions
    newPos = newState([1 4]);
    oldPos = oldState([1 4]);

    % and aim points
    newAim = [nodeX(newIndex);nodeY(newIndex)];
    oldAim = [nodeX(oldIndex);nodeY(oldIndex)];
    
    % distances
    dAimNew = norm(newPos-newAim);
    dAimOld = norm(oldPos-oldAim);
    d2Flown = norm(newPos-oldPos);
    tFlown = 0.15;
    
    % speed
    v = 0.4;
    
    % TD learning gain
    alpha = 1; % set one here and scale outside
    
    % temporal difference update
    newCost = nodeVout(oldIndex) + alpha*(tFlown+dAimNew/v+nodeVin(newIndex) - dAimOld/v-nodeVin(oldIndex));
    
    % absurd for it to go negative
    nodeVout(oldIndex) = max([newCost nodeVout(oldIndex)]);
    
end
